simulink model "sim_modes_data"  (R2014a)
settings: Solver=ode45  StartTime=0.0  StopTime=10.0  RelTol=1e-3
Description:
  | Copyright 2014 The MathWorks, Inc.
settings Model: Creator=smiller  LastModifiedBy=psanghvi
settings DebuggingCC: UnderspecifiedInitializationDetection=Classic  StateNameClashWarn=warning

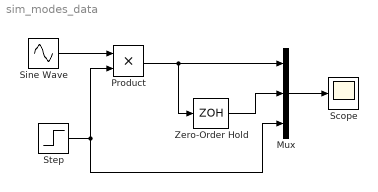
== system sim_modes_data ==
  Mux : Mux  Inputs=3
  Product : Product
  Scope : Scope
      settings: SaveName=SimModesData
  Sine Wave : Sin  Frequency=4*pi/5  SampleTime=0
  Step : Step  Time=5  Before=1  After=0.5  SampleTime=0
  Zero-Order Hold : ZeroOrderHold  SampleTime=0.2
  wires:
  Mux/1 -> Scope/1
  Zero-Order Hold/1 -> Mux/2
  Product/1 -> Zero-Order Hold/1, Mux/1
  Sine Wave/1 -> Product/1
  Step/1 -> Product/2, Mux/3
